simulink model "lead_decreasing_space_gap"  (R2025a)
settings: Solver=VariableStepAuto  StartTime=0.0  StopTime=10.0  RelTol=1e-3
settings Model: Creator=sanborkl  LastModifiedBy=sanborkl

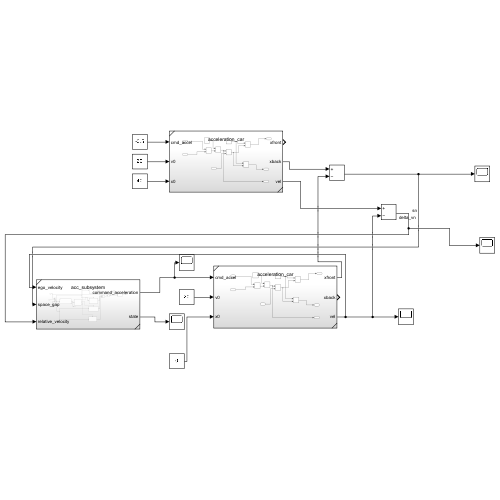
[thumbnail: Simulink's stored preview of the top-level diagram]
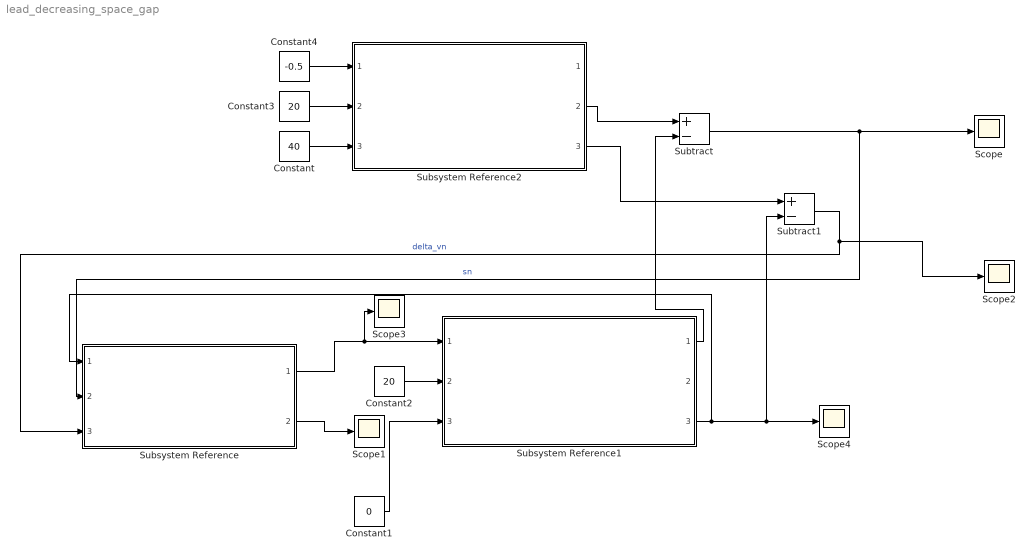
== system lead_decreasing_space_gap ==
  Constant : Constant  Value=40
  Constant1 : Constant  Value=0
  Constant2 : Constant  Value=20
  Constant3 : Constant  Value=20
  Constant4 : Constant  Value=-0.5
  Scope{,1..4} (5 alike) : Scope
      Scope settings: ActiveDisplayYMinimum=-1  ActiveDisplayYMaximum=1
      Scope1 settings: ActiveDisplayYMinimum=-0.12499999999999997  ActiveDisplayYMaximum=1.125  DataLoggingVariableName=ScopeData2
      Scope2 settings: ActiveDisplayYMinimum=-1.2920646047715598  ActiveDisplayYMaximum=1.7202460461415816  DataLoggingVariableName=ScopeData3
      Scope3 settings: ActiveDisplayYMinimum=-3.4431632097936697  ActiveDisplayYMaximum=0.98846888814302758  DataLoggingVariableName=ScopeData4
      Scope4 settings: ActiveDisplayYMinimum=15.489710413072967  ActiveDisplayYMaximum=20.501143287436339
  Subsystem Reference : Subsystem  ReferencedSubsystem=acc_subsystem
  Subsystem Reference1 : Subsystem  ReferencedSubsystem=acceleration_car
  Subsystem Reference2 : Subsystem  ReferencedSubsystem=acceleration_car
  Subtract : Sum  Inputs=+-
  Subtract1 : Sum  Inputs=+-
  wires:
  Subsystem Reference1/3 -> Subsystem Reference/1, Subtract1/2, Scope4/1
  Subtract/1 -> Subsystem Reference/2, Scope/1  "sn"
  Subtract1/1 -> Scope2/1, Subsystem Reference/3  "delta_vn"
  Subsystem Reference2/2 -> Subtract/1
  Subsystem Reference/2 -> Scope1/1
  Constant/1 -> Subsystem Reference2/3
  Constant2/1 -> Subsystem Reference1/2
  Subsystem Reference1/1 -> Subtract/2
  Constant3/1 -> Subsystem Reference2/2
  Subsystem Reference/1 -> Scope3/1, Subsystem Reference1/1
  Subsystem Reference2/3 -> Subtract1/1
  Constant1/1 -> Subsystem Reference1/3
  Constant4/1 -> Subsystem Reference2/1
